simulink model "IP_LQG_Design_Lihao"  (R2024b)
settings: Solver=FixedStepAuto  StartTime=0.0  StopTime=10  FixedStep=0.01  RelTol=1e-3
values from neighbouring files (symbols this model uses):
  A = [0  0   1    0 ... (first row only)    [Init_Setup_LQRArd.m]
  B = [0; 0; mm; nn]    [Init_Setup_LQRArd.m]
  b = 0.00007892    (= 7.892e-05)    [Init_Setup_LQRArd.m]
  c = 0.63    [Init_Setup_LQRArd.m]
  C_lqg = [1 0 0 0 ... (first row only)    [Init_Setup_LQRArd.m]
  g = 9.81    [Init_Setup_LQRArd.m]
  I = 0.0007176    [Init_Setup_LQRArd.m]
  kb = 0.031    [Init_Setup_LQRArd.m]
  KK = lqr(A_nom, B_nom, Q, R)    [Init_Setup_LQRArd.m]
  kt = 0.031    [Init_Setup_LQRArd.m]
  l = input('Longitud del péndulo (m): ')    [Init_Setup_LQRArd.m]
  M = 0.136    [Init_Setup_LQRArd.m]
  m = 0.1    [Init_Setup_LQRArd.m]
  r = 0.006    [Init_Setup_LQRArd.m]
  Rm = 12.5    [Init_Setup_LQRArd.m]
undefined symbols (not defined in the file or in its folder): L, theta0_real, X0_kalman, x0_real
libraries: vrlib x3, simulink x3
settings Model: Creator=jitendra  LastModifiedBy=lihao
settings DataIOCC: ExternalInput=getinputstruct(op_trim1)  InitialState=getstatestruct(op_trim1)  ReturnWorkspaceOutputs=off
settings DebuggingCC: UnconnectedInputMsg=warning  UnconnectedOutputMsg=warning  UnconnectedLineMsg=warning  ArithmeticOperatorsInVariantConditions=warning
settings ModelReferenceCC: EnableRefExpFcnMdlSchedulingChecks=on
settings SFSimCC: SimUseLocalCustomCode=off  CustomCodeUndefinedFunction=UseInterfaceOnly
settings RTWCC: RTWUseLocalCustomCode=off  GPUComputeCapability=3.5

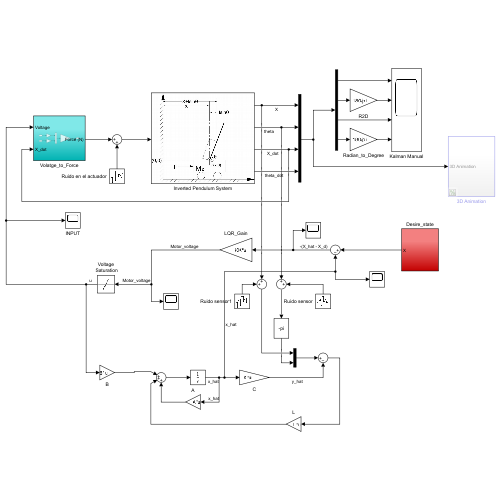
[thumbnail: Simulink's stored preview of the top-level diagram]
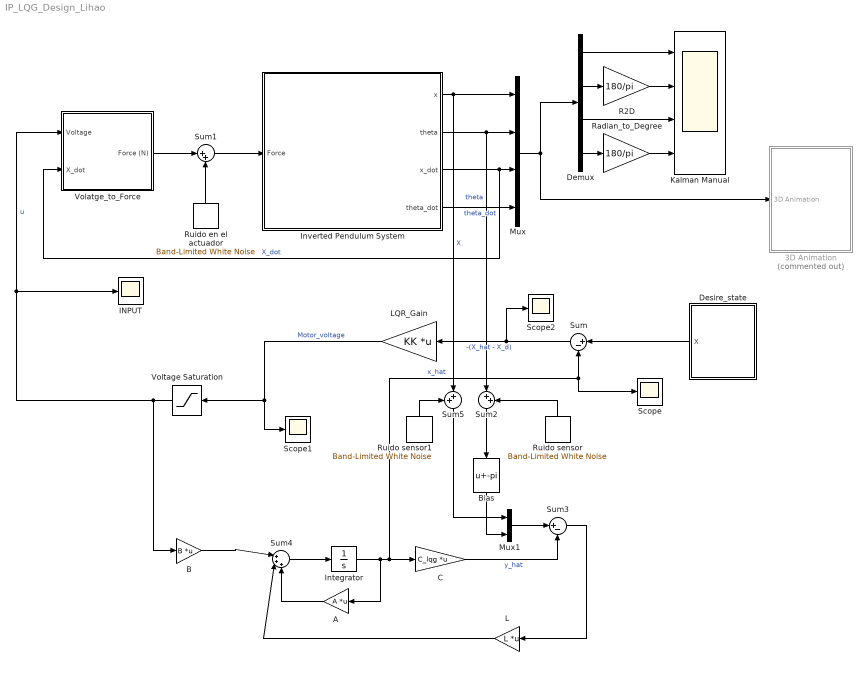
== system IP_LQG_Design_Lihao ==
  3D Animation : Subsystem  Commented=on
  A : Gain  Gain=A  Multiplication=Matrix(K*u)
  B : Gain  Gain=B  Multiplication=Matrix(K*u)
  Bias : Bias  Bias=-pi  SaturateOnIntegerOverflow=off
  C : Gain  Gain=C_lqg  Multiplication=Matrix(K*u)
  Demux : Demux
  Desire_state : Subsystem
  INPUT : Scope
  Integrator : Integrator  InitialCondition=X0_kalman
  Inverted Pendulum System : Subsystem
      mask Display: image('ip_model.png');
  Kalman Manual : Scope  NumInputPorts=4
  L : Gain  Gain=L  Multiplication=Matrix(K*u)
  LQR_Gain : Gain  Gain=KK  Multiplication=Matrix(K*u)
  Mux : Mux
  Mux1 : Mux  Inputs=2
  R2D : Gain  Gain=180/pi
  Radian_to_Degree : Gain  Gain=180/pi
  Ruido en el actuador : simulink/Sources/Band-Limited White Noise  Cov=0  Ts=0.1  seed=[23341]
  Ruido sensor : simulink/Sources/Band-Limited White Noise  Cov=0.0001  Ts=0.1  seed=[23342]
  Ruido sensor1 : simulink/Sources/Band-Limited White Noise  Cov=0.0001  Ts=0.1  seed=[23343]
  Scope : Scope
  Scope1 : Scope
  Scope2 : Scope
  Sum : Sum  Inputs=|+-
  Sum1 : Sum  Inputs=|++
  Sum2 : Sum  Inputs=|++
  Sum3 : Sum  Inputs=|+-
  Sum4 : Sum  Inputs=|+++
  Sum5 : Sum  Inputs=++|
  Volatge_to_Force : Subsystem
  Voltage Saturation : Saturate  UpperLimit=30  LowerLimit=-30
  wires:
  Inverted Pendulum System/3(x_dot) -> Volatge_to_Force/2(X_dot), Mux/3  "X_dot"
  Inverted Pendulum System/2(theta) -> Sum2/1, Mux/2  "theta"
  Inverted Pendulum System/1(x) -> Mux/1, Sum5/2  "X"
  Inverted Pendulum System/4(theta_dot) -> Mux/4  "theta_dot"
  Mux/1 -> Demux/1, 3D Animation/1(3D Animation)
  LQR_Gain/1 -> Scope1/1, Voltage Saturation/1  "Motor_voltage"
  Demux/2 -> R2D/1
  Demux/1 -> Kalman Manual/1
  Demux/3 -> Kalman Manual/3
  Demux/4 -> Radian_to_Degree/1
  R2D/1 -> Kalman Manual/2
  Radian_to_Degree/1 -> Kalman Manual/4
  Integrator/1 -> Scope/1, Sum/2, C/1, A/1  "x_hat"
  Mux1/1 -> Sum3/1
  C/1 -> Sum3/2  "y_hat"
  Sum3/1 -> L/1
  B/1 -> Sum4/1
  A/1 -> Sum4/3
  L/1 -> Sum4/2
  Sum4/1 -> Integrator/1
  Sum/1 -> LQR_Gain/1, Scope2/1  "-(X_hat - X_d)"
  Desire_state/1(X) -> Sum/1
  Voltage Saturation/1 -> B/1, INPUT/1, Volatge_to_Force/1(Voltage)  "u"
  Ruido en el actuador/1 -> Sum1/2
  Sum1/1 -> Inverted Pendulum System/1(Force)
  Volatge_to_Force/1(Force (N)) -> Sum1/1
  Ruido sensor/1 -> Sum2/2
  Sum5/1 -> Mux1/1
  Ruido sensor1/1 -> Sum5/1
  Sum2/1 -> Bias/1
  Bias/1 -> Mux1/2

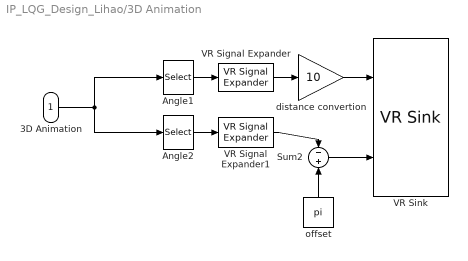
== system IP_LQG_Design_Lihao/3D Animation ==
  3D Animation : Inport
  Angle1 : Selector  InputPortWidth=4  IndexOptions=Index vector (dialog)  Indices=[1]  OutputSizes=1
  Angle2 : Selector  InputPortWidth=4  IndexOptions=Index vector (dialog)  Indices=[2]  OutputSizes=1
  Sum2 : Sum  Inputs=-|+
  VR Signal Expander : vrlib/VR Signal Expander  outwidth=3  outidx=[1]
  VR Signal Expander1 : vrlib/VR Signal Expander  outwidth=4  outidx=[4]
  VR Sink : vrlib/VR Sink  InstantiateOnLoad=on  SampleTime=0.02  ViewEnable=on  RemoteChange=off  RemoteView=off  FieldsWritten=cart.translation.3.1.1.double#joint.rotation.4.1.1.double  WorldFileName=Inverted_pendulum12.wrl  AutoView=off  VideoDimensions=[]  AllowVariableSize=off
  distance convertion : Gain  Gain=10
  offset : Constant  Value=pi
  wires:
  VR Signal Expander/1 -> distance convertion/1
  3D Animation/1 -> Angle2/1, Angle1/1
  Angle1/1 -> VR Signal Expander/1
  Angle2/1 -> VR Signal Expander1/1
  offset/1 -> Sum2/2
  Sum2/1 -> VR Sink/2
  VR Signal Expander1/1 -> Sum2/1
  distance convertion/1 -> VR Sink/1

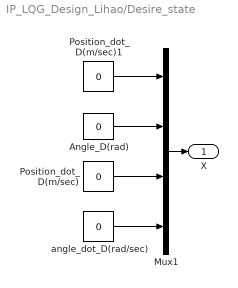
== system IP_LQG_Design_Lihao/Desire_state ==
  Angle_D(rad) : Constant  Value=0
  Mux1 : Mux
  Position_dot_D(m/sec) : Constant  Value=0
  Position_dot_D(m/sec)1 : Constant  Value=0
  angle_dot_D(rad/sec) : Constant  Value=0
  X : Outport  VectorParamsAs1DForOutWhenUnconnected=off
  wires:
  Mux1/1 -> X/1
  Position_dot_D(m/sec)/1 -> Mux1/3
  angle_dot_D(rad/sec)/1 -> Mux1/4
  Angle_D(rad)/1 -> Mux1/2
  Position_dot_D(m/sec)1/1 -> Mux1/1

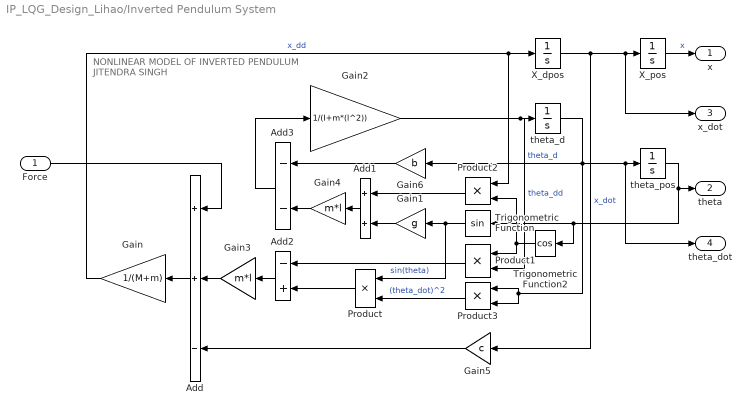
== system IP_LQG_Design_Lihao/Inverted Pendulum System ==
  note: NONLINEAR MODEL OF
      | INVERTED PENDULUM
      | JITENDRA SINGH
  Force : Inport
  Add : Sum  Inputs=++-
  Add1 : Sum
  Add2 : Sum  Inputs=-+
  Add3 : Sum  Inputs=--
  Gain : Gain  Gain=1/(M+m)
  Gain1 : Gain  Gain=g
  Gain2 : Gain  Gain=1/(I+m*(l^2))
  Gain3 : Gain  Gain=m*l
  Gain4 : Gain  Gain=m*l
  Gain5 : Gain  Gain=c
  Gain6 : Gain  Gain=b
  Product{,1..3} (4 alike) : Product
  Trigonometric Function : Trigonometry
  Trigonometric Function2 : Trigonometry  Operator=cos
  X_dpos : Integrator
  X_pos : Integrator  InitialCondition=x0_real
  theta_d : Integrator
  theta_pos : Integrator  InitialCondition=theta0_real
  x : Outport  VectorParamsAs1DForOutWhenUnconnected=off
  theta : Outport  Port=2  VectorParamsAs1DForOutWhenUnconnected=off
  x_dot : Outport  Port=3  VectorParamsAs1DForOutWhenUnconnected=off
  theta_dot : Outport  Port=4  VectorParamsAs1DForOutWhenUnconnected=off
  wires:
  Gain5/1 -> Add/3
  Add2/1 -> Gain3/1
  Add3/1 -> Gain2/1
  Trigonometric Function2/1 -> Product2/2, Product1/1
  Trigonometric Function/1 -> Product/1, Gain1/1  "sin(theta)"
  Gain3/1 -> Add/2
  theta_d/1 -> Product3/2, Product3/1, Gain6/1, theta_dot/1, theta_pos/1  "theta_d"
  Product2/1 -> Add1/1
  Product/1 -> Add2/2
  Gain4/1 -> Add3/2
  Product3/1 -> Product/2  "(theta_dot)^2"
  X_pos/1 -> x/1  "x"
  Product1/1 -> Add2/1
  Gain/1 -> X_dpos/1, Product2/1  "x_dd"
  Add/1 -> Gain/1
  Gain2/1 -> Product1/2, theta_d/1  "theta_dd"
  Gain6/1 -> Add3/1
  theta_pos/1 -> Trigonometric Function2/1, Trigonometric Function/1, theta/1
  Force/1 -> Add/1
  Gain1/1 -> Add1/2
  X_dpos/1 -> x_dot/1, X_pos/1, Gain5/1  "x_dot"
  Add1/1 -> Gain4/1

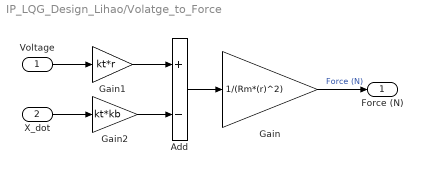
== system IP_LQG_Design_Lihao/Volatge_to_Force ==
  Voltage : Inport
  X_dot : Inport  Port=2
  Add : Sum  Inputs=+-
  Gain : Gain  Gain=1/(Rm*(r)^2)
  Gain1 : Gain  Gain=kt*r
  Gain2 : Gain  Gain=kt*kb
  Force (N) : Outport  VectorParamsAs1DForOutWhenUnconnected=off
  wires:
  Gain1/1 -> Add/1
  Gain2/1 -> Add/2
  Voltage/1 -> Gain1/1
  Gain/1 -> Force (N)/1  "Force (N)"
  X_dot/1 -> Gain2/1
  Add/1 -> Gain/1
